simulink model "SerialTransmit_Test"  (R2017b)
settings: Solver=FixedStepAuto  StartTime=0.0  StopTime=10.0  FixedStep=0.001  RelTol=1e-3  EnableMultiTasking=on
libraries: etargetslib x1, frdmk64flib x1
settings Model: ExtModeTrigDuration=5  Creator=brydoa1  LastModifiedBy=Daniel
settings OptimizationCC: PassReuseOutputArgsAs=Individual arguments  MaxStackSize=64
settings DebuggingCC: ParameterTunabilityLossMsg=error
settings HardwareCC: ProdBitPerPointer=32  ProdBitPerSizeT=32  ProdBitPerPtrDiffT=32  ProdLargestAtomicInteger=Long  ProdLargestAtomicFloat=Double  ProdWordSize=32  ProdHWDeviceType=ARM Compatible->ARM Cortex
settings SFSimCC: MATLABDynamicMemAlloc=off
settings RTWCC: SystemTargetFile=ert.tlc  HardwareBoard=NXP FRDM-K64F  TemplateMakefile=ert_default_tmf  GenerateReport=on  Toolchain=GNU Tools for ARM Embedded Processors  IncludeHyperlinkInReport=on  LaunchReport=on  GenerateTraceInfo=on  GenerateTraceReport=on  GenerateTraceReportSl=on  GenerateTraceReportSf=on  GenerateTraceReportEml=on
settings CodeAppCC: ForceParamTrailComments=on  IgnoreCustomStorageClasses=off  OperatorAnnotations=on  SimulinkDataObjDesc=on  SFDataObjDesc=on  InsertBlockDesc=on

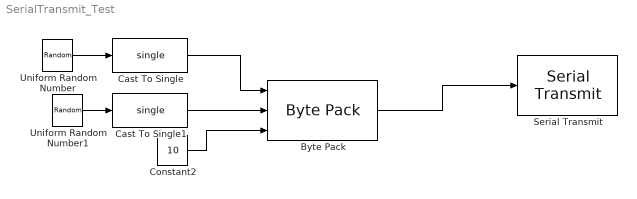
== system SerialTransmit_Test ==
  Byte Pack : etargetslib/Byte Pack  datatypes={'single','single','uint8'}  byteAlign=1
  Cast To Single : DataTypeConversion  OutDataTypeStr=single
  Cast To Single1 : DataTypeConversion  OutDataTypeStr=single
  Constant2 : Constant  Value=10  OutDataTypeStr=uint8  SampleTime=0.001
  Serial Transmit : frdmk64flib/Serial Transmit  SCIModule=0  Baudrate=uint32(9600)  Parity=None  StopBits=1  HardwareFlowControl=None  ByteOrder=LittleEndian  BlockingMode=on  OutputStatus=off
      settings: SourceProductName=Simulink Coder Support Package for NXP FRDM-K64F Board
  Uniform Random Number : UniformRandomNumber  Minimum=-4  Maximum=4  Seed=123  SampleTime=0.001
  Uniform Random Number1 : UniformRandomNumber  Minimum=-4  Maximum=4  Seed=456  SampleTime=0.001
  wires:
  Byte Pack/1 -> Serial Transmit/1
  Cast To Single/1 -> Byte Pack/1
  Cast To Single1/1 -> Byte Pack/2
  Constant2/1 -> Byte Pack/3
  Uniform Random Number/1 -> Cast To Single/1
  Uniform Random Number1/1 -> Cast To Single1/1
